simulink model "simulacion_con_f"  (R2021a)
settings: Solver=VariableStepAuto  StartTime=0.0  StopTime=10.0  RelTol=1e-3
settings Model: Creator=franc  LastModifiedBy=franc

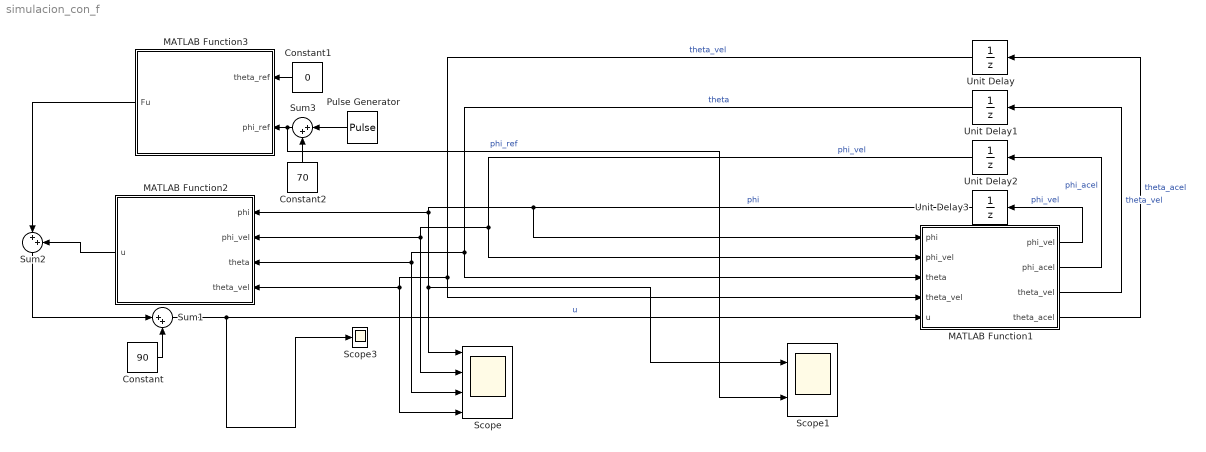
== system simulacion_con_f ==
  Constant : Constant  Value=90
  Constant1 : Constant  Value=0
  Constant2 : Constant  Value=70
  MATLAB Function1 : MATLAB Function  TreatAsAtomicUnit=on
  MATLAB Function2 : MATLAB Function  TreatAsAtomicUnit=on
  MATLAB Function3 : MATLAB Function  TreatAsAtomicUnit=on
  Pulse Generator : DiscretePulseGenerator  PulseType=Time based  Amplitude=60  Period=10  PulseWidth=50  PhaseDelay=2
  Scope : Scope  NumInputPorts=4
  Scope1 : Scope  NumInputPorts=2
  Scope3 : Scope
  Sum1 : Sum  Inputs=|++
  Sum2 : Sum  Inputs=|++
  Sum3 : Sum  Inputs=|++
  Unit Delay : UnitDelay  SampleTime=0.01  HasFrameUpgradeWarning=on
  Unit Delay1 : UnitDelay  SampleTime=0.01  HasFrameUpgradeWarning=on
  Unit Delay2 : UnitDelay  SampleTime=0.01  HasFrameUpgradeWarning=on
  Unit Delay3 : UnitDelay  InitialCondition=90  SampleTime=0.01  HasFrameUpgradeWarning=on
  wires:
  MATLAB Function1/1(phi_vel) -> Unit Delay3/1  "phi_vel"
  MATLAB Function1/2(phi_acel) -> Unit Delay2/1  "phi_acel"
  Unit Delay2/1 -> MATLAB Function2/2(phi_vel), Scope/2, MATLAB Function1/2("phi_vel ")  "phi_vel"
  MATLAB Function1/3(theta_vel) -> Unit Delay1/1  "theta_vel"
  MATLAB Function1/4(theta_acel) -> Unit Delay/1  "theta_acel"
  Unit Delay3/1 -> Scope/1, Scope1/1, MATLAB Function2/1(phi), MATLAB Function1/1(phi)  "phi"
  Unit Delay1/1 -> MATLAB Function2/3(theta), Scope/3, MATLAB Function1/3(theta)  "theta"
  Sum1/1 -> Scope3/1, MATLAB Function1/5(u)  "u"
  Constant/1 -> Sum1/2
  Unit Delay/1 -> MATLAB Function1/4("theta_vel "), Scope/4, MATLAB Function2/4(theta_vel)  "theta_vel"
  MATLAB Function3/1(Fu) -> Sum2/1
  MATLAB Function2/1(u) -> Sum2/2
  Sum2/1 -> Sum1/1
  Constant1/1 -> MATLAB Function3/1(theta_ref)
  Sum3/1 -> Scope1/2, MATLAB Function3/2(phi_ref)  "phi_ref"
  Pulse Generator/1 -> Sum3/1
  Constant2/1 -> Sum3/2

== matlab function simulacion_con_f/MATLAB Function1 ==
  data: phi input; phi_vel input; theta input; theta_vel input; u input; phi_vel output; phi_acel output; theta_vel output; theta_acel output
function [phi_vel,phi_acel,theta_vel,theta_acel] = fcn(phi,phi_vel,theta,theta_vel,u)

Ad = [
    1.0000    0.0100         0         0;
   -0.5765    0.9895   -2.1322   -0.2132;
         0         0    1.0000    0.0100;
         0         0   -2.5000    0.7500;
];
   
Bd = [
         0;
  2.132250;
         0;
  2.500000
];

x  = [theta theta_vel phi phi_vel];
x_dot = Ad * x' + Bd * u;
theta_vel = x_dot(1);
theta_acel = x_dot(2);
phi_vel = x_dot(3);
phi_acel = x_dot(4);

== matlab function simulacion_con_f/MATLAB Function2 ==
  data: phi input; phi_vel input; theta input; theta_vel input; u output
function u = fcn(phi,phi_vel,theta,theta_vel)
    K = [-0.5, 0.001, 0.7, -0.005];
    u = K(1) * theta + K(2) * theta_vel + K(3) * (phi - 90) + K(4) * phi_vel;

== matlab function simulacion_con_f/MATLAB Function3 ==
  data: theta_ref input; phi_ref input; Fu output
function Fu = fcn(theta_ref, phi_ref)
    F = [0, 0.3];
    Fu = F(1) * theta_ref + F(2) * (phi_ref-90);
